simulink model "mconversion6"  (Simulink 8.0)
settings: Solver=FixedStepDiscrete  StartTime=0.0  StopTime=10.0  RelTol=1e-3
settings Model: Creator=awarlock  LastModifiedBy=htu  ExtModeAutoUpdateStatusClock=off
settings DataIOCC: SignalLoggingSaveFormat=ModelDataLogs  SaveOutput=off  SaveTime=off  SignalLoggingName=logsOut
settings OptimizationCC: InlineParams=on  InlineInvariantSignals=on  InitFltsAndDblsToZero=on
settings DebuggingCC: SaveWithParameterizedLinksMsg=none  CheckExecutionContextPreStartOutputMsg=on  CheckExecutionContextRuntimeOutputMsg=on  SignalResolutionControl=TryResolveAllWithWarning  MultiTaskDSMMsg=warning  MultiTaskCondExecSysMsg=none
settings RTWCC: IncludeERTFirstTime=on
settings GRTTargetCC: TargetFcnLib=ansi_tfl_tmw.mat  CombineOutputUpdateFcns=off  GRTInterface=on

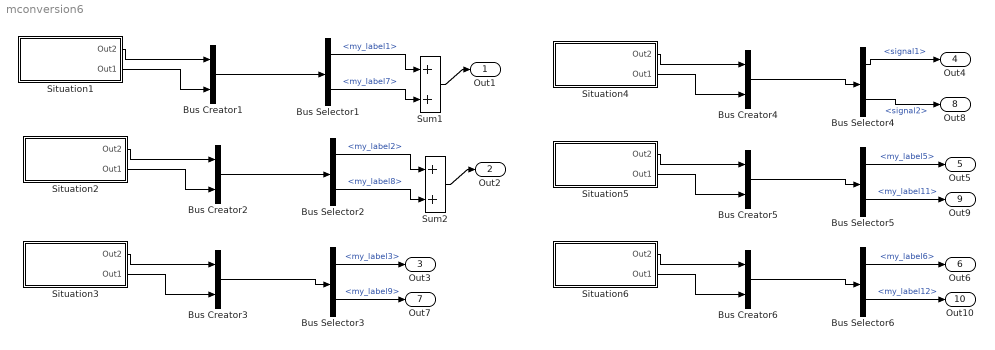
== system mconversion6 ==
  Bus Creator{1..6} (6 alike) : BusCreator  DialogController=Simulink.DDGSource_Bus  Inputs=2
  Bus Selector1 : BusSelector  DialogController=Simulink.DDGSource_Bus  OutputSignals=my_label1,my_label7
  Bus Selector2 : BusSelector  DialogController=Simulink.DDGSource_Bus  OutputSignals=my_label2,my_label8
  Bus Selector3 : BusSelector  DialogController=Simulink.DDGSource_Bus  OutputSignals=my_label3,my_label9
  Bus Selector4 : BusSelector  DialogController=Simulink.DDGSource_Bus  OutputSignals=signal1,signal2
  Bus Selector5 : BusSelector  DialogController=Simulink.DDGSource_Bus  OutputSignals=my_label5,my_label11
  Bus Selector6 : BusSelector  DialogController=Simulink.DDGSource_Bus  OutputSignals=my_label6,my_label12
  Situation1 : Subsystem  TreatAsAtomicUnit=on
  Situation2 : Subsystem  TreatAsAtomicUnit=on
  Situation3 : Subsystem  TreatAsAtomicUnit=on
  Situation4 : Subsystem  TreatAsAtomicUnit=on
  Situation5 : Subsystem  TreatAsAtomicUnit=on
  Situation6 : Subsystem  TreatAsAtomicUnit=on
  Sum1 : Sum  Inputs=|++
  Sum2 : Sum  Inputs=|++
  Out1 : Outport
  Out2 : Outport  Port=2
  Out3 : Outport  Port=3
  Out4 : Outport  Port=4
  Out5 : Outport  Port=5
  Out6 : Outport  Port=6
  Out7 : Outport  Port=7
  Out8 : Outport  Port=8
  Out9 : Outport  Port=9
  Out10 : Outport  Port=10
  wires:
  Situation1/1(Out2) -> Bus Creator1/1
  Bus Creator1/1 -> Bus Selector1/1
  Situation1/2(Out1) -> Bus Creator1/2
  Bus Selector1/1 -> Sum1/1  "<my_label1>"
  Bus Selector1/2 -> Sum1/2  "<my_label7>"
  Sum1/1 -> Out1/1
  Situation2/1(Out2) -> Bus Creator2/1
  Bus Creator2/1 -> Bus Selector2/1
  Situation2/2(Out1) -> Bus Creator2/2
  Bus Selector2/1 -> Sum2/1  "<my_label2>"
  Bus Selector2/2 -> Sum2/2  "<my_label8>"
  Sum2/1 -> Out2/1
  Situation3/1(Out2) -> Bus Creator3/1
  Bus Creator3/1 -> Bus Selector3/1
  Situation4/1(Out2) -> Bus Creator4/1
  Bus Creator4/1 -> Bus Selector4/1
  Situation5/1(Out2) -> Bus Creator5/1
  Bus Creator5/1 -> Bus Selector5/1
  Situation6/1(Out2) -> Bus Creator6/1
  Bus Creator6/1 -> Bus Selector6/1
  Bus Selector3/1 -> Out3/1  "<my_label3>"
  Bus Selector4/1 -> Out4/1  "<signal1>"
  Bus Selector5/1 -> Out5/1  "<my_label5>"
  Bus Selector6/1 -> Out6/1  "<my_label6>"
  Situation3/2(Out1) -> Bus Creator3/2
  Bus Selector3/2 -> Out7/1  "<my_label9>"
  Situation4/2(Out1) -> Bus Creator4/2
  Bus Selector4/2 -> Out8/1  "<signal2>"
  Situation5/2(Out1) -> Bus Creator5/2
  Bus Selector5/2 -> Out9/1  "<my_label11>"
  Situation6/2(Out1) -> Bus Creator6/2
  Bus Selector6/2 -> Out10/1  "<my_label12>"

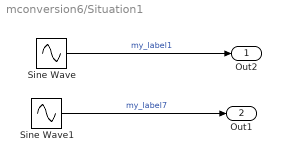
== system mconversion6/Situation1 ==
  Sine Wave : Sin  SampleTime=0.1
  Sine Wave1 : Sin  SampleTime=0.1
  Out2 : Outport
  Out1 : Outport  Port=2
  wires:
  Sine Wave/1 -> Out2/1  "my_label1"
  Sine Wave1/1 -> Out1/1  "my_label7"

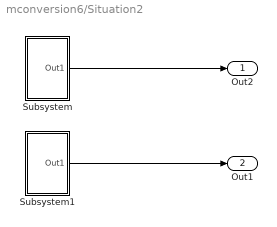
== system mconversion6/Situation2 ==
  Subsystem : Subsystem
  Subsystem1 : Subsystem
  Out2 : Outport
  Out1 : Outport  Port=2
  wires:
  Subsystem/1(Out1) -> Out2/1
  Subsystem1/1(Out1) -> Out1/1

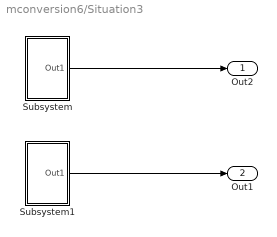
== system mconversion6/Situation3 ==
  Subsystem : Subsystem
  Subsystem1 : Subsystem
  Out2 : Outport
  Out1 : Outport  Port=2
  wires:
  Subsystem/1(Out1) -> Out2/1
  Subsystem1/1(Out1) -> Out1/1

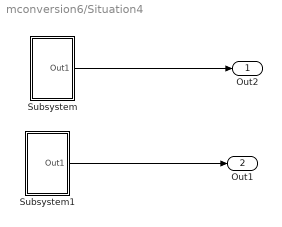
== system mconversion6/Situation4 ==
  Subsystem : Subsystem
  Subsystem1 : Subsystem
  Out2 : Outport
  Out1 : Outport  Port=2
  wires:
  Subsystem/1(Out1) -> Out2/1
  Subsystem1/1(Out1) -> Out1/1

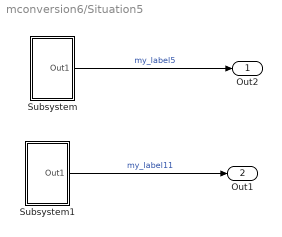
== system mconversion6/Situation5 ==
  Subsystem : Subsystem
  Subsystem1 : Subsystem
  Out2 : Outport
  Out1 : Outport  Port=2
  wires:
  Subsystem/1(Out1) -> Out2/1  "my_label5"
  Subsystem1/1(Out1) -> Out1/1  "my_label11"

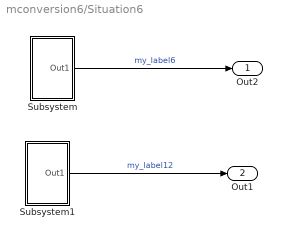
== system mconversion6/Situation6 ==
  Subsystem : Subsystem
  Subsystem1 : Subsystem
  Out2 : Outport
  Out1 : Outport  Port=2
  wires:
  Subsystem/1(Out1) -> Out2/1  "my_label6"
  Subsystem1/1(Out1) -> Out1/1  "my_label12"

== system mconversion6/Situation2/Subsystem ==
  Sine Wave : Sin  SampleTime=0.1
  Out1 : Outport
  wires:
  Sine Wave/1 -> Out1/1  "my_label2"

== system mconversion6/Situation2/Subsystem1 ==
  Sine Wave : Sin  SampleTime=0.1
  Out1 : Outport
  wires:
  Sine Wave/1 -> Out1/1  "my_label8"

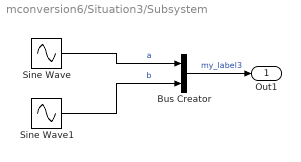
== system mconversion6/Situation3/Subsystem ==
  Bus Creator : BusCreator  DialogController=Simulink.DDGSource_Bus  Inputs=2
  Sine Wave : Sin  SampleTime=0.1
  Sine Wave1 : Sin  SampleTime=0.1
  Out1 : Outport
  wires:
  Sine Wave/1 -> Bus Creator/1  "a"
  Bus Creator/1 -> Out1/1  "my_label3"
  Sine Wave1/1 -> Bus Creator/2  "b"

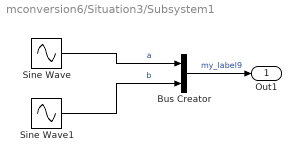
== system mconversion6/Situation3/Subsystem1 ==
  Bus Creator : BusCreator  DialogController=Simulink.DDGSource_Bus  Inputs=2
  Sine Wave : Sin  SampleTime=0.1
  Sine Wave1 : Sin  SampleTime=0.1
  Out1 : Outport
  wires:
  Sine Wave1/1 -> Bus Creator/2  "b"
  Bus Creator/1 -> Out1/1  "my_label9"
  Sine Wave/1 -> Bus Creator/1  "a"

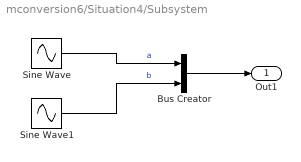
== system mconversion6/Situation4/Subsystem ==
  Bus Creator : BusCreator  DialogController=Simulink.DDGSource_Bus  Inputs=2
  Sine Wave : Sin  SampleTime=0.1
  Sine Wave1 : Sin  SampleTime=0.1
  Out1 : Outport
  wires:
  Sine Wave1/1 -> Bus Creator/2  "b"
  Bus Creator/1 -> Out1/1
  Sine Wave/1 -> Bus Creator/1  "a"

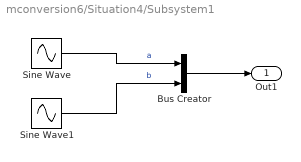
== system mconversion6/Situation4/Subsystem1 ==
  Bus Creator : BusCreator  DialogController=Simulink.DDGSource_Bus  Inputs=2
  Sine Wave : Sin  SampleTime=0.1
  Sine Wave1 : Sin  SampleTime=0.1
  Out1 : Outport
  wires:
  Sine Wave/1 -> Bus Creator/1  "a"
  Bus Creator/1 -> Out1/1
  Sine Wave1/1 -> Bus Creator/2  "b"

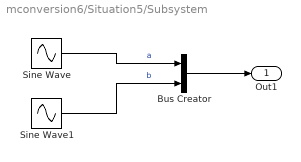
== system mconversion6/Situation5/Subsystem ==
  Bus Creator : BusCreator  DialogController=Simulink.DDGSource_Bus  Inputs=2
  Sine Wave : Sin  SampleTime=0.1
  Sine Wave1 : Sin  SampleTime=0.1
  Out1 : Outport
  wires:
  Sine Wave/1 -> Bus Creator/1  "a"
  Bus Creator/1 -> Out1/1
  Sine Wave1/1 -> Bus Creator/2  "b"

== system mconversion6/Situation5/Subsystem1 ==
  Bus Creator : BusCreator  DialogController=Simulink.DDGSource_Bus  Inputs=2
  Sine Wave : Sin  SampleTime=0.1
  Sine Wave1 : Sin  SampleTime=0.1
  Out1 : Outport
  wires:
  Sine Wave1/1 -> Bus Creator/2  "b"
  Bus Creator/1 -> Out1/1
  Sine Wave/1 -> Bus Creator/1  "a"

== system mconversion6/Situation6/Subsystem ==
  Bus Creator : BusCreator  DialogController=Simulink.DDGSource_Bus  Inputs=2
  Sine Wave : Sin  SampleTime=0.1
  Sine Wave1 : Sin  SampleTime=0.1
  Out1 : Outport
  wires:
  Sine Wave1/1 -> Bus Creator/2  "b"
  Bus Creator/1 -> Out1/1  "z"
  Sine Wave/1 -> Bus Creator/1  "a"

== system mconversion6/Situation6/Subsystem1 ==
  Bus Creator : BusCreator  DialogController=Simulink.DDGSource_Bus  Inputs=2
  Sine Wave : Sin  SampleTime=0.1
  Sine Wave1 : Sin  SampleTime=0.1
  Out1 : Outport
  wires:
  Sine Wave/1 -> Bus Creator/1  "a"
  Bus Creator/1 -> Out1/1  "z"
  Sine Wave1/1 -> Bus Creator/2  "b"
